simulink model "AM_Modulation"  (R2012b)
settings: Solver=FixedStepDiscrete  StartTime=0.0  StopTime=10.0  RelTol=1e-3
settings Model: Creator=Ahmad  LastModifiedBy=Ahmad

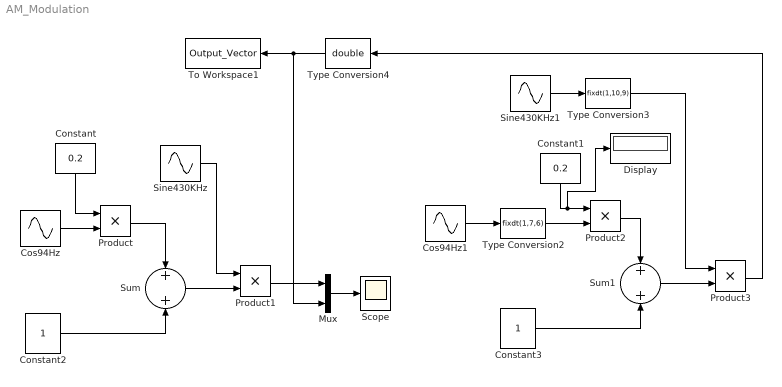
== system AM_Modulation ==
  Constant : Constant  Value=0.2  VectorParams1D=off  OutDataTypeStr=double  SampleTime=1/100e6
  Constant1 : Constant  Value=0.2  VectorParams1D=off  OutDataTypeStr=fixdt(1,8,7)  SampleTime=1/100e6
  Constant2 : Constant  VectorParams1D=off  OutDataTypeStr=double  SampleTime=1/100e6
  Constant3 : Constant  VectorParams1D=off  OutDataTypeStr=fixdt(1,2,0)  SampleTime=1/100e6
  Cos94Hz : Sin  Frequency=2*pi*94  Phase=pi/2  SampleTime=1/100e6
  Cos94Hz1 : Sin  Frequency=2*pi*94  Phase=pi/2  SampleTime=1/100e6
  Display : Display
  Mux : Mux  Inputs=2
  Product{,1..3} (4 alike) : Product  RndMeth=Zero
  Scope : Scope
      settings: TimeRange=7.000000000000062e-05  YMin=-3  YMax=4
  Sine430KHz : Sin  Frequency=2*pi*430e3  SampleTime=1/100e6
  Sine430KHz1 : Sin  Frequency=2*pi*430e3  SampleTime=1/100e6
  Sum : Sum  Inputs=+|+
  Sum1 : Sum  Inputs=+|+
  To Workspace1 : ToWorkspace  VariableName=Output_Vector  SampleTime=-1  SaveFormat=Timeseries
  Type Conversion2 : DataTypeConversion  OutDataTypeStr=fixdt(1,7,6)  SaturateOnIntegerOverflow=on
  Type Conversion3 : DataTypeConversion  OutDataTypeStr=fixdt(1,10,9)  RndMeth=Round  SaturateOnIntegerOverflow=on
  Type Conversion4 : DataTypeConversion  OutDataTypeStr=double
  wires:
  Constant/1 -> Product/1
  Cos94Hz/1 -> Product/2
  Product/1 -> Sum/1
  Mux/1 -> Scope/1
  Type Conversion4/1 -> Mux/2, To Workspace1/1
  Product3/1 -> Type Conversion4/1
  Constant2/1 -> Sum/2
  Sum/1 -> Product1/2
  Sine430KHz/1 -> Product1/1
  Product1/1 -> Mux/1
  Constant1/1 -> Display/1, Product2/1
  Cos94Hz1/1 -> Type Conversion2/1
  Product2/1 -> Sum1/1
  Constant3/1 -> Sum1/2
  Sum1/1 -> Product3/2
  Sine430KHz1/1 -> Type Conversion3/1
  Type Conversion2/1 -> Product2/2
  Type Conversion3/1 -> Product3/1
